simulink model "main"  (R2016a)
settings: Solver=FixedStepAuto  StartTime=0.0  StopTime=inf  FixedStep=0.008  RelTol=1e-3
model workspace: external: MATLAB File initialize_variables_kuramoto.m (data not in the file)
values from neighbouring files (symbols this model uses):
  Angle_offset = [Offset_st, Offset_dev, Offset_rot]    [initialize_variables_kuramoto.m]
  frequency_multiplier = 1    [initialize_variables_kuramoto.m]
  learning_switch = 0    [initialize_variables_matsuoka.m]
  max_dev = 30    [initialize_variables_kuramoto.m]    (also in initialize_variables_matsuoka.m)
  max_rot = 60    [initialize_variables_kuramoto.m]    (also in initialize_variables_matsuoka.m = 90)
  max_stroke = 180    [initialize_variables_kuramoto.m]    (also in initialize_variables_matsuoka.m = 90)
  Offset_st = 0 * gain_st    (= 0)    [initialize_variables_kuramoto.m]
  param_init = [0,0,0,0,0,0 ... (first row only)    [cpg_param_sets.m]    (also in initialize_variables_matsuoka.m)
  param_list = zeros([7,length(Re)*length(A_star)])    [initialize_variables_kuramoto.m]
  step_time = 0.005    [initialize_variables_kuramoto.m]
  w_init = [0 -1.5 0 0 0 0 ... (first row only)    [cpg_param_sets.m]    (also in initialize_variables_matsuoka.m = [0 -2 0 0 -0.1 0)
undefined symbols (not defined in the file or in its folder): frequency, IO3xx, Offset_dev_rot, V
libraries: slrtlib x13, speedgoatlib_fpga x7, simulink x5, powerlib_meascontrol x2
(part 1 of 2)
settings Model: Creator=cedric  LastModifiedBy=kqp5516
settings SolverCC: EnableConcurrentExecution=on
settings DataIOCC: SaveFormat=StructureWithTime  SignalLogging=off  DSMLogging=off  SaveTime=off
settings OptimizationCC: BlockReduction=off  OptimizeBlockIOStorage=off  BufferReuse=off  GlobalBufferReuse=off  ExpressionFolding=off  LocalBlockOutputs=off
settings DebuggingCC: UnderspecifiedInitializationDetection=Classic  MergeDetectMultiDrivingBlocksExec=none  UnconnectedInputMsg=none  UnconnectedOutputMsg=none  UnconnectedLineMsg=none  SFUnexpectedBacktrackingDiag=error  SFNoUnconditionalDefaultTransitionDiag=error
settings HardwareCC: ProdBitPerPointer=32  ProdLargestAtomicFloat=None  ProdWordSize=32  ProdHWDeviceType=Generic->32-bit x86 compatible
settings ModelReferenceCC: PropagateSignalLabelsOutOfModel=off
settings RTWCC: SystemTargetFile=slrt.tlc  TemplateMakefile=slrt_default_tmf  Description=Simulink Real-Time  RTWCompilerOptimization=on
settings SimulinkRealTimeCC: RL32LogTETModifier=off  xPCisModelTimeout=off  xPCModelTimeoutSecs=20
settings ConfigComp: CovMetricSettings=dwe  CovHtmlReporting=off  CovSaveCumulativeToWorkspaceVar=off  CovSaveSingleToWorkspaceVar=off  CovExternalEMLEnable=on

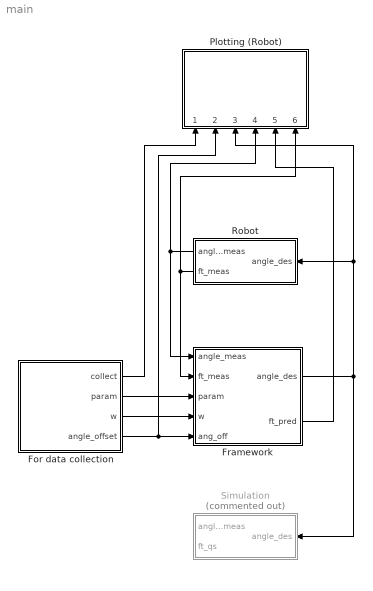
== system main ==
  For data collection : Subsystem
  Framework : Subsystem
  Plotting (Robot) : Subsystem
  Robot : Subsystem
  Simulation : Subsystem  Commented=on
  wires:
  Robot/2(ft_meas) -> Framework/2(ft_meas), Plotting (Robot)/6(ft_meas)
  Robot/1(angle_meas) -> Framework/1(angle_meas), Plotting (Robot)/4(angle_meas)
  Framework/2(ft_pred) -> Plotting (Robot)/5(ft_pred)
  For data collection/4(angle_offset) -> Framework/5(ang_off), Plotting (Robot)/2(angle_offset)
  For data collection/2(param) -> Framework/3(param)
  For data collection/3(w) -> Framework/4(w)
  For data collection/1(collect) -> Plotting (Robot)/1(collect)
  Framework/1(angle_des) -> Plotting (Robot)/3(angle_des), Robot/1(angle_des), Simulation/1(angle_des)

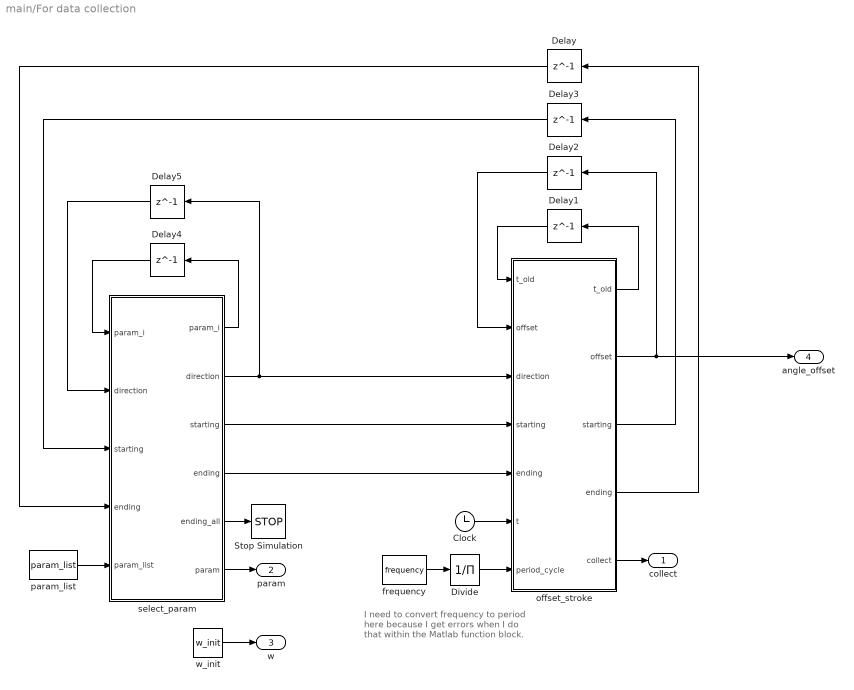
== system main/For data collection ==
  note: I need to convert frequency to period here because I get errors when I do that within the Matlab function block.
  Clock : Clock
  Delay : Delay  DelayLength=1  InitialCondition=0
  Delay1 : Delay  DelayLength=1  InitialCondition=0
  Delay2 : Delay  DelayLength=1  InitialCondition=zeros(3,1)
  Delay3 : Delay  DelayLength=1  InitialCondition=1
  Delay4 : Delay  DelayLength=1  InitialCondition=1
  Delay5 : Delay  DelayLength=1  InitialCondition=1
  Divide : Product  Inputs=/
  Stop Simulation : Stop
  frequency : Constant  Value=frequency
  offset_stroke : MATLAB Function  TreatAsAtomicUnit=on
  param_list : Constant  Value=param_list
  select_param : MATLAB Function  TreatAsAtomicUnit=on
  w_init : Constant  Value=w_init
  collect : Outport
  param : Outport  Port=2
  w : Outport  Port=3
  angle_offset : Outport  Port=4
  wires:
  offset_stroke/2(offset) -> angle_offset/1, Delay2/1
  offset_stroke/4(ending) -> Delay/1
  offset_stroke/1(t_old) -> Delay1/1
  Delay1/1 -> offset_stroke/1("t_old ")
  Delay2/1 -> offset_stroke/2("offset ")
  offset_stroke/3(starting) -> Delay3/1
  Delay3/1 -> select_param/3("starting ")
  Delay/1 -> select_param/4("ending ")
  select_param/3(starting) -> offset_stroke/4("starting ")
  select_param/4(ending) -> offset_stroke/5("ending ")
  select_param/1(param_i) -> Delay4/1
  Delay4/1 -> select_param/1("param_i ")
  select_param/2(direction) -> Delay5/1, offset_stroke/3(direction)
  Delay5/1 -> select_param/2("direction ")
  select_param/5(ending_all) -> Stop Simulation/1
  select_param/6(param) -> param/1
  param_list/1 -> select_param/5(param_list)
  Clock/1 -> offset_stroke/6(t)
  frequency/1 -> Divide/1
  Divide/1 -> offset_stroke/7(period_cycle)
  offset_stroke/5(collect) -> collect/1
  w_init/1 -> w/1

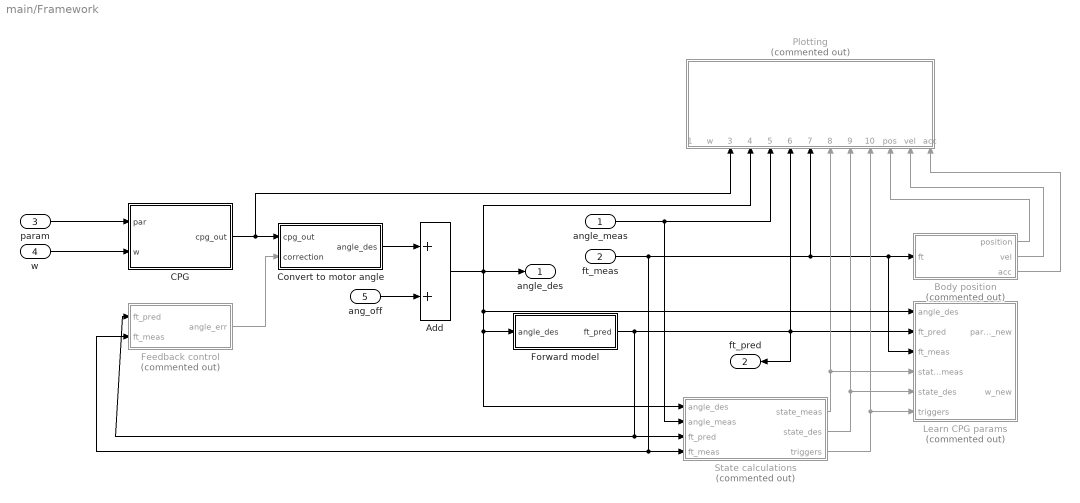
== system main/Framework ==
  angle_meas : Inport
  ft_meas : Inport  Port=2
  param : Inport  Port=3
  w : Inport  Port=4
  ang_off : Inport  Port=5
  Add : Sum
  Body position : Subsystem  Commented=on
  CPG : Subsystem
  Convert to motor angle : Subsystem
  Feedback control : Subsystem  Commented=on
  Forward model : Subsystem
  Learn CPG params : Subsystem  Commented=on
  Plotting : Subsystem  Commented=on
  State calculations : Subsystem  Commented=on
  angle_des : Outport
  ft_pred : Outport  Port=2
  wires:
  CPG/1(cpg_out) -> Plotting/3(cpg_out), Convert to motor angle/1(cpg_out)
  ft_meas/1 -> Plotting/7(ft_meas), Learn CPG params/3(ft_meas), Body position/1(ft), State calculations/4(ft_meas), Feedback control/2(ft_meas)
  State calculations/2(state_des) -> Plotting/9(state_des), Learn CPG params/5(state_des)
  Forward model/1(ft_pred) -> Feedback control/1(ft_pred), State calculations/3(ft_pred), ft_pred/1, Learn CPG params/2(ft_pred), Plotting/6(ft_pred)
  Feedback control/1(angle_err) -> Convert to motor angle/2(correction)
  State calculations/3(triggers) -> Plotting/10(triggers), Learn CPG params/6(triggers)
  Body position/2(vel) -> Plotting/12(vel)
  Body position/1(position) -> Plotting/11(pos)
  Body position/3(acc) -> Plotting/13(acc)
  State calculations/1(state_meas) -> Plotting/8(state_meas), Learn CPG params/4(state_meas)
  angle_meas/1 -> State calculations/2(angle_meas), Plotting/5(angle_meas)
  Convert to motor angle/1(angle_des) -> Add/1
  param/1 -> CPG/1(par)
  w/1 -> CPG/2(w)
  ang_off/1 -> Add/2
  Add/1 -> angle_des/1, Plotting/4(angle_des), State calculations/1(angle_des), Forward model/1(angle_des), Learn CPG params/1(angle_des)

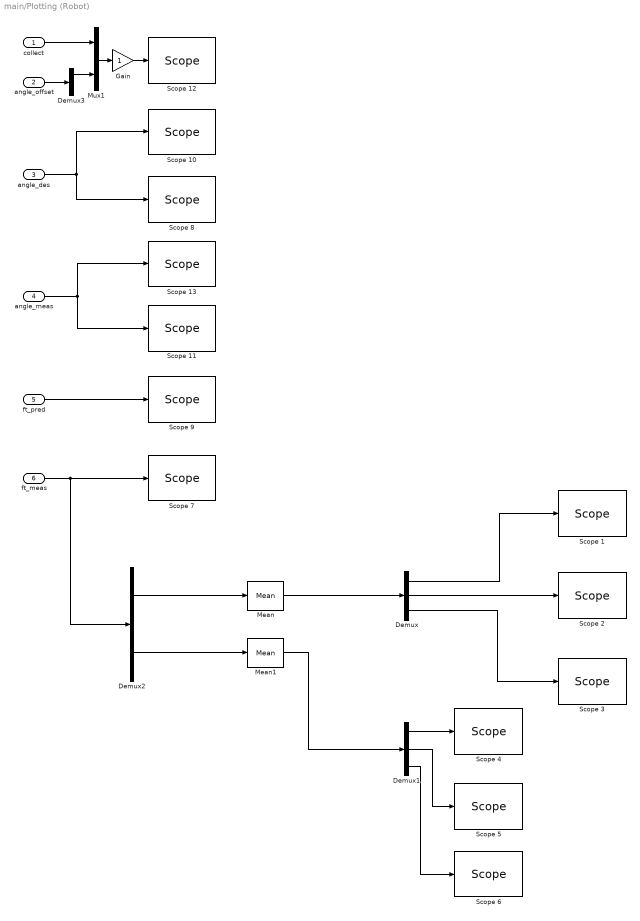
== system main/Plotting (Robot) ==
  collect : Inport
  angle_offset : Inport  Port=2
  angle_des : Inport  Port=3
  angle_meas : Inport  Port=4
  ft_pred : Inport  Port=5
  ft_meas : Inport  Port=6
  Demux : Demux  Outputs=3
  Demux1 : Demux  Outputs=3
  Demux2 : Demux  Outputs=2
  Demux3 : Demux  Outputs=3
  Gain : Gain
  Mean : powerlib_meascontrol/Measurements/Mean  Freq=10  Vinit=0  Ts=0.008
  Mean1 : powerlib_meascontrol/Measurements/Mean  Freq=10  Vinit=0  Ts=0.008
  Mux1 : Mux  Inputs=2
  Scope 1 : slrtlib/Displays and Logging/Scope   scopeno=1  scopetype=Target  autostart=on  viewmode=Graphical rolling  formatstr='%15.6f'  grid=on  ylimits=[0,0]  nosamples=1000  noprepostsamples=0  interleave=5  triggermode=FreeRun  triggersignal=1  trigsignalfromport=off  triggerlevel=0.5  triggerslope=Either  triggerscope=1  triggersample=11000  filename=data.dat  mode=Lazy  writesize=512  autorestart=off  dynamicfilemode=off  maxwritefilesize=512*1024^2
  Scope 10 : slrtlib/Displays and Logging/Scope   scopeno=10  scopetype=File  autostart=on  viewmode=Graphical rolling  formatstr='%15.6f'  grid=on  ylimits=[0,0]  nosamples=10000  noprepostsamples=0  interleave=1  triggermode=FreeRun  triggersignal=1  trigsignalfromport=off  triggerlevel=0.5  triggerslope=Rising  triggerscope=1  triggersample=0  filename=ANGDES_<%>.dat  mode=Lazy  writesize=512  autorestart=on  dynamicfilemode=on  maxwritefilesize=512*1024^2
  Scope 11 : slrtlib/Displays and Logging/Scope   scopeno=11  scopetype=File  autostart=on  viewmode=Graphical rolling  formatstr='%15.6f'  grid=on  ylimits=[0,0]  nosamples=10000  noprepostsamples=0  interleave=1  triggermode=FreeRun  triggersignal=1  trigsignalfromport=off  triggerlevel=0.5  triggerslope=Rising  triggerscope=1  triggersample=0  filename=ANGMEA_<%>.dat  mode=Lazy  writesize=512  autorestart=on  dynamicfilemode=on  maxwritefilesize=512*1024^2
  Scope 12 : slrtlib/Displays and Logging/Scope   scopeno=12  scopetype=File  autostart=on  viewmode=Graphical rolling  formatstr='%15.6f'  grid=on  ylimits=[0,0]  nosamples=10000  noprepostsamples=0  interleave=1  triggermode=FreeRun  triggersignal=1  trigsignalfromport=off  triggerlevel=0.5  triggerslope=Rising  triggerscope=1  triggersample=0  filename=ANGOFF_<%>.dat  mode=Lazy  writesize=512  autorestart=on  dynamicfilemode=on  maxwritefilesize=512*1024^2
  Scope 13 : slrtlib/Displays and Logging/Scope   scopeno=13  scopetype=Target  autostart=on  viewmode=Graphical rolling  formatstr='%15.6f'  grid=on  ylimits=[0,0]  nosamples=1000  noprepostsamples=0  interleave=5  triggermode=FreeRun  triggersignal=1  trigsignalfromport=off  triggerlevel=0.5  triggerslope=Rising  triggerscope=1  triggersample=0  filename=data.dat  mode=Lazy  writesize=512  autorestart=off  dynamicfilemode=off  maxwritefilesize=512*1024^2
  Scope 2 : slrtlib/Displays and Logging/Scope   scopeno=2  scopetype=Target  autostart=on  viewmode=Graphical rolling  formatstr='%15.6f'  grid=on  ylimits=[0,0]  nosamples=1000  noprepostsamples=0  interleave=5  triggermode=FreeRun  triggersignal=1  trigsignalfromport=off  triggerlevel=0.5  triggerslope=Either  triggerscope=1  triggersample=0  filename=data.dat  mode=Lazy  writesize=512  autorestart=off  dynamicfilemode=off  maxwritefilesize=512*1024^2
  Scope 3 : slrtlib/Displays and Logging/Scope   scopeno=3  scopetype=Target  autostart=on  viewmode=Graphical rolling  formatstr='%15.6f'  grid=on  ylimits=[0,0]  nosamples=1000  noprepostsamples=0  interleave=5  triggermode=FreeRun  triggersignal=1  trigsignalfromport=off  triggerlevel=0.5  triggerslope=Rising  triggerscope=1  triggersample=0  filename=data.dat  mode=Lazy  writesize=512  autorestart=off  dynamicfilemode=off  maxwritefilesize=512*1024^2
  Scope 4 : slrtlib/Displays and Logging/Scope   scopeno=4  scopetype=Target  autostart=on  viewmode=Graphical rolling  formatstr='%15.6f'  grid=on  ylimits=[0,0]  nosamples=1000  noprepostsamples=0  interleave=5  triggermode=FreeRun  triggersignal=1  trigsignalfromport=off  triggerlevel=0.5  triggerslope=Rising  triggerscope=1  triggersample=0  filename=data.dat  mode=Lazy  writesize=512  autorestart=off  dynamicfilemode=off  maxwritefilesize=512*1024^2
  Scope 5 : slrtlib/Displays and Logging/Scope   scopeno=5  scopetype=Target  autostart=on  viewmode=Graphical rolling  formatstr='%15.6f'  grid=on  ylimits=[0,0]  nosamples=1000  noprepostsamples=0  interleave=5  triggermode=Software triggering  triggersignal=1  trigsignalfromport=off  triggerlevel=0.5  triggerslope=Rising  triggerscope=1  triggersample=0  filename=data.dat  mode=Lazy  writesize=512  autorestart=off  dynamicfilemode=off  maxwritefilesize=512*1024^2
  Scope 6 : slrtlib/Displays and Logging/Scope   scopeno=6  scopetype=Target  autostart=on  viewmode=Graphical rolling  formatstr='%15.6f'  grid=on  ylimits=[0,0]  nosamples=1000  noprepostsamples=0  interleave=5  triggermode=FreeRun  triggersignal=1  trigsignalfromport=off  triggerlevel=0.5  triggerslope=Rising  triggerscope=1  triggersample=0  filename=data.dat  mode=Lazy  writesize=512  autorestart=off  dynamicfilemode=off  maxwritefilesize=512*1024^2
  Scope 7 : slrtlib/Displays and Logging/Scope   scopeno=7  scopetype=File  autostart=on  viewmode=Graphical rolling  formatstr='%15.6f'  grid=on  ylimits=[0,0]  nosamples=10000  noprepostsamples=0  interleave=1  triggermode=FreeRun  triggersignal=1  trigsignalfromport=off  triggerlevel=0.5  triggerslope=Rising  triggerscope=1  triggersample=0  filename=FTMEA_<%>.dat  mode=Lazy  writesize=512  autorestart=on  dynamicfilemode=on  maxwritefilesize=512*1024^2
  Scope 8 : slrtlib/Displays and Logging/Scope   scopeno=8  scopetype=Target  autostart=on  viewmode=Graphical rolling  formatstr='%15.6f'  grid=on  ylimits=[0,0]  nosamples=1000  noprepostsamples=0  interleave=5  triggermode=FreeRun  triggersignal=1  trigsignalfromport=off  triggerlevel=0.5  triggerslope=Rising  triggerscope=1  triggersample=0  filename=data.dat  mode=Lazy  writesize=512  autorestart=off  dynamicfilemode=off  maxwritefilesize=512*1024^2
  Scope 9 : slrtlib/Displays and Logging/Scope   scopeno=9  scopetype=File  autostart=on  viewmode=Graphical rolling  formatstr='%15.6f'  grid=on  ylimits=[0,0]  nosamples=10000  noprepostsamples=0  interleave=1  triggermode=FreeRun  triggersignal=1  trigsignalfromport=off  triggerlevel=0.5  triggerslope=Rising  triggerscope=1  triggersample=0  filename=FTPRE_<%>.dat  mode=Lazy  writesize=512  autorestart=on  dynamicfilemode=on  maxwritefilesize=512*1024^2
  wires:
  ft_meas/1 -> Demux2/1, Scope 7/1
  Mean/1 -> Demux/1
  Mean1/1 -> Demux1/1
  Demux1/1 -> Scope 4/1
  Demux1/2 -> Scope 5/1
  Demux1/3 -> Scope 6/1
  Demux/1 -> Scope 1/1
  Demux/2 -> Scope 2/1
  Demux/3 -> Scope 3/1
  Demux2/1 -> Mean/1
  Demux2/2 -> Mean1/1
  angle_des/1 -> Scope 10/1, Scope 8/1
  angle_meas/1 -> Scope 13/1, Scope 11/1
  ft_pred/1 -> Scope 9/1
  collect/1 -> Mux1/1
  angle_offset/1 -> Demux3/1
  Demux3/1 -> Mux1/2
  Mux1/1 -> Gain/1
  Gain/1 -> Scope 12/1

== system main/Robot ==
  angle_des : Inport
  Analog Force Signal : Subsystem
  Control : Subsystem
  Serial Setup : speedgoatlib_fpga/Serial/Serial Setup  id=1  channel=[1 6]  bitrate_configuration=Simple  bitrate=[1000000]  bitrate_effective=[1e6, 1e6]  bitrate_error=[0, 0]  base_clock=[75000000, 75000000]  divider=[5, 5]  cpr=[1, 1]  tcr=[15, 15]  parity=No parity  nb_data_bits=[8]  nb_stop_bits=[1]  rs485_half_duplex=on  board=IO323  pciSlot=-1
  Setup : speedgoatlib_fpga/Setup/Setup  board=IO323  id=1  frontIO=None  rearIO=IO3xx-22  bitstreamFile=speedgoat_IO323_22_CI_01532  ProgSpiFlash=off  ProgBPIFlash=off  pciSlot=-1  PullRPort0=pull-up 3.3V  VioPort0=3.3V  PullRPort1=pull-up 3.3V  VioPort1=3.3V  PullRPort2=pull-up 3.3V  VioPort2=3.3V  PullRPort3=pull-up 3.3V  VioPort3=3.3V  PullRPort4=pull-up 3.3V  VioPort4=3.3V  PullRPort5=pull-up 3.3V  VioPort5=3.3V  PullRPort6=pull-up 3.3V  VioPort6=3.3V  PullRPort15=pull-up 3.3V  PullRPort31=pull-up 3.3V  PullRPort47=pull-up 3.3V  PullRPort63=pull-up 3.3V
  angle_meas : Outport
  ft_meas : Outport  Port=2
  wires:
  angle_des/1 -> Control/1(reference)
  Control/1(ang_meas) -> angle_meas/1
  Analog Force Signal/1(ft) -> ft_meas/1

== system main/Simulation ==
  angle_des : Inport  PortDimensions=3
  Add : Sum
  Band-Limited White Noise : simulink/Sources/Band-Limited White Noise  Commented=on  Cov=[0.0001,0.0001,0.0001]  Ts=0.008  seed=[23341,438,1376]
  Demux : Demux  Commented=on  Outputs=3
  QS Model : Subsystem
  Scope : Scope  Commented=on  NumInputPorts=3
  angle_meas : Outport
  ft_qs : Outport  Port=2
  wires:
  angle_des/1 -> Add/1, angle_meas/1
  QS Model/1(ft_qs) -> ft_qs/1
  Add/1 -> QS Model/1(angle_des)
  Band-Limited White Noise/1 -> Add/2, Demux/1
  Demux/1 -> Scope/1
  Demux/2 -> Scope/2
  Demux/3 -> Scope/3

== system main/Framework/Body position ==
  ft : Inport  PortDimensions=6
  Equations of motion : MATLAB Function  TreatAsAtomicUnit=on
  Integrator : Integrator  InitialCondition=zeros(3,1)
  Integrator1 : Integrator  InitialCondition=zeros(3,1)
  position : Outport
  vel : Outport  Port=2
  acc : Outport  Port=3
  wires:
  ft/1 -> Equations of motion/1(ft)
  Equations of motion/1(acc) -> acc/1, Integrator/1
  Integrator/1 -> Integrator1/1, vel/1
  Integrator1/1 -> position/1

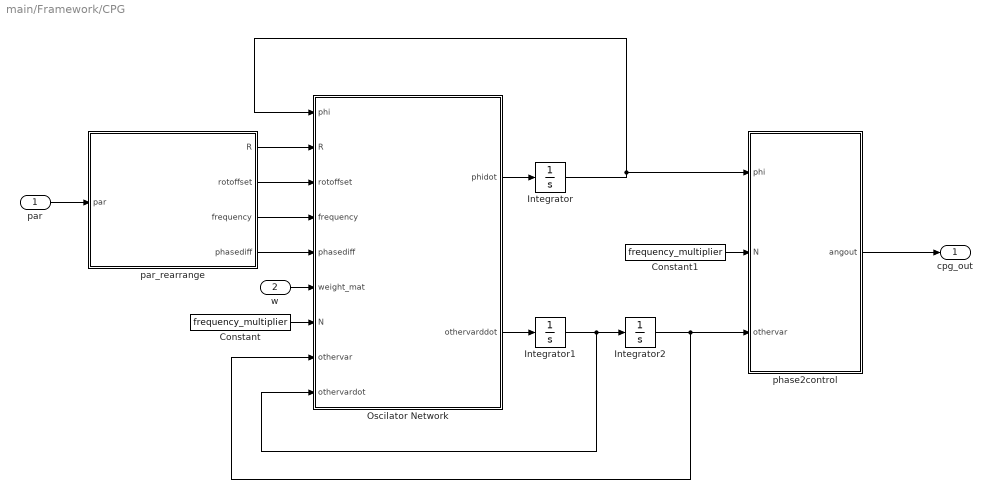
== system main/Framework/CPG ==
  par : Inport
  w : Inport  Port=2
  Constant : Constant  Value=frequency_multiplier
  Constant1 : Constant  Value=frequency_multiplier
  Integrator : Integrator
  Integrator1 : Integrator
  Integrator2 : Integrator
  Oscilator Network : MATLAB Function  TreatAsAtomicUnit=on
  par_rearrange : MATLAB Function  TreatAsAtomicUnit=on
  phase2control : MATLAB Function  TreatAsAtomicUnit=on
  cpg_out : Outport
  wires:
  par/1 -> par_rearrange/1(par)
  Oscilator Network/1(phidot) -> Integrator/1
  par_rearrange/1(R) -> Oscilator Network/2(R)
  Oscilator Network/2(othervarddot) -> Integrator1/1
  Integrator1/1 -> Integrator2/1, Oscilator Network/9(othervardot)
  Integrator2/1 -> Oscilator Network/8(othervar), phase2control/3(othervar)
  par_rearrange/3(frequency) -> Oscilator Network/4(frequency)
  par_rearrange/4(phasediff) -> Oscilator Network/5(phasediff)
  phase2control/1(angout) -> cpg_out/1
  par_rearrange/2(rotoffset) -> Oscilator Network/3(rotoffset)
  Integrator/1 -> Oscilator Network/1(phi), phase2control/1(phi)
  Constant/1 -> Oscilator Network/7(N)
  Constant1/1 -> phase2control/2(N)
  w/1 -> Oscilator Network/6(weight_mat)

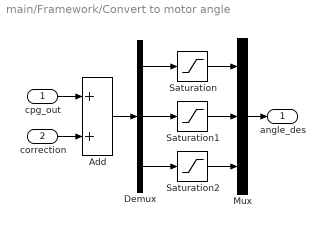
== system main/Framework/Convert to motor angle ==
  cpg_out : Inport  Interpolate=off
  correction : Inport  Port=2
  Add : Sum
  Demux : Demux  Outputs=3
  Mux : Mux  Inputs=3
  Saturation : Saturate  UpperLimit=max_stroke  LowerLimit=-max_stroke
  Saturation1 : Saturate  UpperLimit=max_dev  LowerLimit=-max_dev
  Saturation2 : Saturate  UpperLimit=max_rot  LowerLimit=-max_rot
  angle_des : Outport
  wires:
  Mux/1 -> angle_des/1
  Demux/2 -> Saturation1/1
  Demux/3 -> Saturation2/1
  Demux/1 -> Saturation/1
  Saturation/1 -> Mux/1
  Saturation2/1 -> Mux/3
  Saturation1/1 -> Mux/2
  correction/1 -> Add/2
  cpg_out/1 -> Add/1
  Add/1 -> Demux/1

== system main/Framework/Feedback control ==
  ft_pred : Inport
  ft_meas : Inport  Port=2
  Delay2 : Delay  DelayLength=1
  Delay3 : Delay  DelayLength=1
  MATLAB Function : MATLAB Function  TreatAsAtomicUnit=on
  angle_err : Outport
  wires:
  ft_meas/1 -> Delay2/1
  ft_pred/1 -> Delay3/1
  MATLAB Function/1(angle_correction) -> angle_err/1
  Delay2/1 -> MATLAB Function/2(ft_meas)
  Delay3/1 -> MATLAB Function/1(ft_pred)

== system main/Framework/Forward model ==
  angle_des : Inport
  QS Model : Subsystem
  ft_pred : Outport
  wires:
  angle_des/1 -> QS Model/1(angle_des)
  QS Model/1(ft_qs) -> ft_pred/1

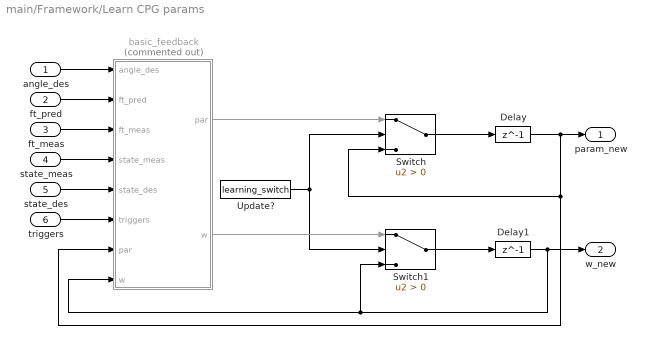
== system main/Framework/Learn CPG params ==
  angle_des : Inport  PortDimensions=3
  ft_pred : Inport  Port=2  PortDimensions=6
  ft_meas : Inport  Port=3  PortDimensions=6
  state_meas : Inport  Port=4
  state_des : Inport  Port=5
  triggers : Inport  Port=6
  Delay : Delay  DelayLength=1  InitialCondition=param_init
  Delay1 : Delay  DelayLength=1  InitialCondition=w_init
  Switch : Switch  Criteria=u2 > Threshold
  Switch1 : Switch  Criteria=u2 > Threshold
  Update? : Constant  Value=learning_switch
  basic_feedback : MATLAB Function  Commented=on  TreatAsAtomicUnit=on
  param_new : Outport
  w_new : Outport  Port=2
  wires:
  ft_meas/1 -> basic_feedback/3(ft_meas)
  ft_pred/1 -> basic_feedback/2(ft_pred)
  angle_des/1 -> basic_feedback/1(angle_des)
  Update?/1 -> Switch/2, Switch1/2
  Switch/1 -> Delay/1
  basic_feedback/1(par) -> Switch/1
  basic_feedback/2(w) -> Switch1/1
  Switch1/1 -> Delay1/1
  triggers/1 -> basic_feedback/6(triggers)
  state_meas/1 -> basic_feedback/4(state_meas)
  state_des/1 -> basic_feedback/5(state_des)
  Delay/1 -> Switch/3, basic_feedback/7("par "), param_new/1
  Delay1/1 -> Switch1/3, basic_feedback/8("w "), w_new/1

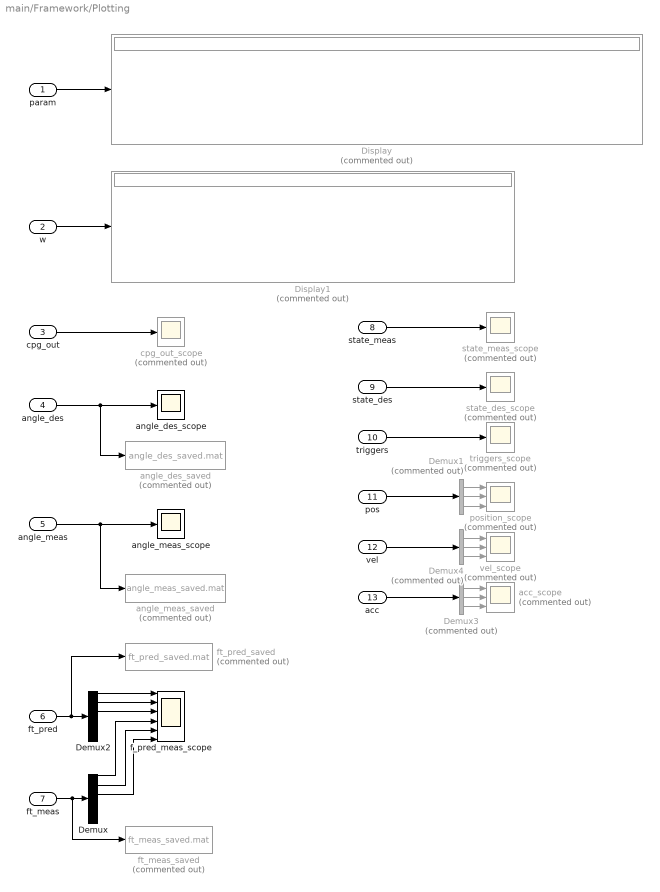
== system main/Framework/Plotting ==
  param : Inport
  w : Inport  Port=2
  cpg_out : Inport  Port=3
  angle_des : Inport  Port=4
  angle_meas : Inport  Port=5
  ft_pred : Inport  Port=6
  ft_meas : Inport  Port=7
  state_meas : Inport  Port=8
  state_des : Inport  Port=9
  triggers : Inport  Port=10
  pos : Inport  Port=11
  vel : Inport  Port=12
  acc : Inport  Port=13
  Demux : Demux  Outputs=6
  Demux1 : Demux  Commented=on  Outputs=3
  Demux2 : Demux  Outputs=6
  Demux3 : Demux  Commented=on  Outputs=3
  Demux4 : Demux  Commented=on  Outputs=3
  Display : Display  Commented=on
  Display1 : Display  Commented=on
  acc_scope : Scope  Commented=on  NumInputPorts=3
  angle_des_saved : ToFile  Commented=on  Filename=angle_des_saved.mat  MatrixName=angle_des_saved
  angle_des_scope : Scope
  angle_meas_saved : ToFile  Commented=on  Filename=angle_meas_saved.mat  MatrixName=angle_meas_saved
  angle_meas_scope : Scope
  cpg_out_scope : Scope  Commented=on
  f_pred_meas_scope : Scope  NumInputPorts=6
  ft_meas_saved : ToFile  Commented=on  Filename=ft_meas_saved.mat  MatrixName=ft_meas_saved
  ft_pred_saved : ToFile  Commented=on  Filename=ft_pred_saved.mat  MatrixName=ft_pred_saved  SaveFormat=Timeseries
  position_scope : Scope  Commented=on  NumInputPorts=3
  state_des_scope : Scope  Commented=on
  state_meas_scope : Scope  Commented=on
  triggers_scope : Scope  Commented=on
  vel_scope : Scope  Commented=on  NumInputPorts=3
  wires:
  Demux1/1 -> position_scope/1
  Demux1/2 -> position_scope/2
  Demux1/3 -> position_scope/3
  Demux3/1 -> acc_scope/1
  Demux3/2 -> acc_scope/2
  Demux3/3 -> acc_scope/3
  Demux4/1 -> vel_scope/1
  Demux4/2 -> vel_scope/2
  Demux4/3 -> vel_scope/3
  pos/1 -> Demux1/1
  vel/1 -> Demux4/1
  acc/1 -> Demux3/1
  ft_meas/1 -> ft_meas_saved/1, Demux/1
  ft_pred/1 -> ft_pred_saved/1, Demux2/1
  cpg_out/1 -> cpg_out_scope/1
  angle_meas/1 -> angle_meas_saved/1, angle_meas_scope/1
  angle_des/1 -> angle_des_saved/1, angle_des_scope/1
  triggers/1 -> triggers_scope/1
  state_meas/1 -> state_meas_scope/1
  param/1 -> Display/1
  w/1 -> Display1/1
  state_des/1 -> state_des_scope/1
  Demux2/1 -> f_pred_meas_scope/1
  Demux2/2 -> f_pred_meas_scope/2
  Demux2/3 -> f_pred_meas_scope/3
  Demux/1 -> f_pred_meas_scope/4
  Demux/2 -> f_pred_meas_scope/5
  Demux/3 -> f_pred_meas_scope/6

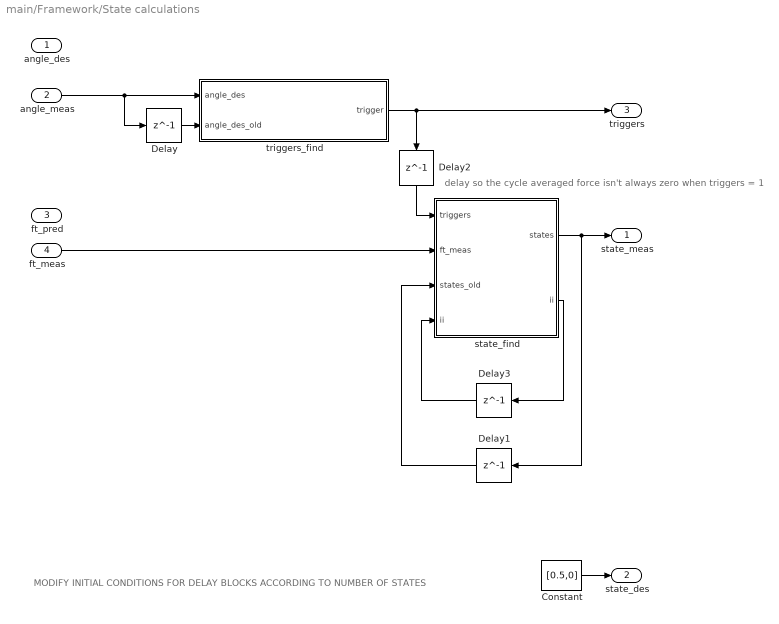
== system main/Framework/State calculations ==
  note: MODIFY INITIAL CONDITIONS FOR DELAY BLOCKS ACCORDING TO NUMBER OF STATES
  note: delay so the cycle averaged force isn't always zero when triggers = 1
  angle_des : Inport
  angle_meas : Inport  Port=2
  ft_pred : Inport  Port=3
  ft_meas : Inport  Port=4
  Constant : Constant  Value=[0.5,0]
  Delay : Delay  DelayLength=1
  Delay1 : Delay  DelayLength=1  InitialCondition=zeros(2,1)
  Delay2 : Delay  DelayLength=1  InitialCondition=zeros(2,1)
  Delay3 : Delay  DelayLength=1  InitialCondition=zeros(2,1)
  state_find : MATLAB Function  TreatAsAtomicUnit=on
  triggers_find : MATLAB Function  TreatAsAtomicUnit=on
  state_meas : Outport
  state_des : Outport  Port=2
  triggers : Outport  Port=3
  wires:
  angle_meas/1 -> Delay/1, triggers_find/1(angle_des)
  Delay/1 -> triggers_find/2(angle_des_old)
  triggers_find/1(trigger) -> triggers/1, Delay2/1
  state_find/1(states) -> Delay1/1, state_meas/1
  Delay1/1 -> state_find/3(states_old)
  ft_meas/1 -> state_find/2(ft_meas)
  Constant/1 -> state_des/1
  Delay2/1 -> state_find/1(triggers)
  state_find/2(ii) -> Delay3/1
  Delay3/1 -> state_find/4("ii ")

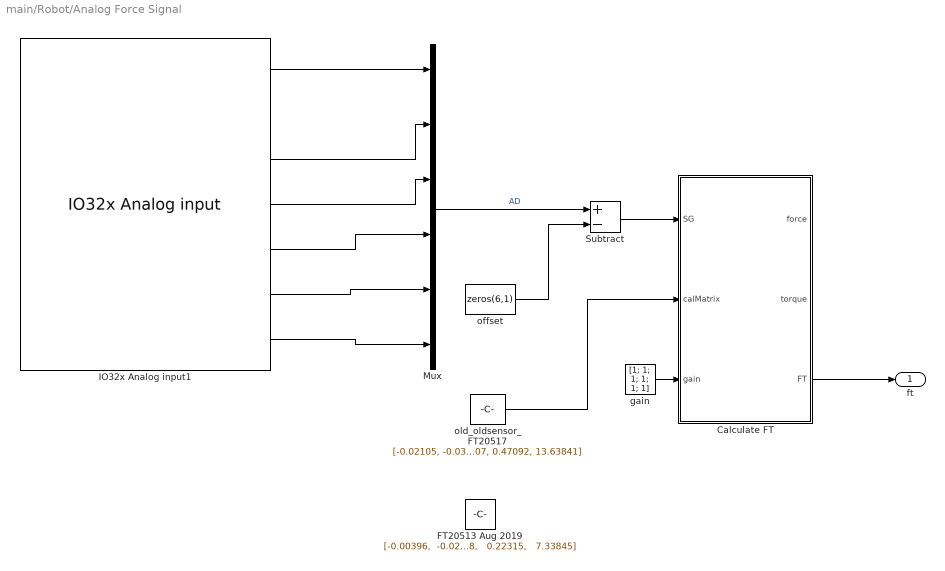
== system main/Robot/Analog Force Signal ==
  Calculate FT : MATLAB Function  TreatAsAtomicUnit=on
  FT20513 Aug 2019 : Constant  Value="[-0.00396,  -0.02626,  -0.00148,  -1.65041,   0.05372,   1.61165;-0.00147,   2.05926,  -0.01141,  -0.98505,  -0.01508,  -0.91035; 1.88736,  -0.01982,   1.94791,  -0.03636,   1.85673,  -0.02132;-0.06688,  12.60494,  10.47872,  -6.15582, -10.64754,  -5.52308; -11.71646,   0.24827,   6.66712,   9.99714,   6.01967,  -9.86076;0.06228,   7.36314,  -0.02169,   7.00298,   0.22315,   7.33845]"  VectorParams1D=off
  IO32x Analog input1 : speedgoatlib_fpga/Analog IO/IO32x Analog input  id=1  pciSlot=-1  board=IO323  ts=step_time  ADC1_chan=[]  ADC1_range=± 5.12 [V]  ADC1_diff=Differential  ADC1_Trigger=Initiator  ADC1_Seq=on  ADC2_chan=[]  ADC2_range=± 5.12 [V]  ADC2_diff=Differential  ADC2_Trigger=Initiator  ADC2_Seq=on  ADC3_chan=[1,2,3,4]  ADC3_range=± 5.12 [V]  ADC3_diff=Differential  ADC3_Trigger=Initiator  ADC3_Seq=on  ADC4_chan=[1,2,3]  ADC4_range=± 5.12 [V]  ADC4_diff=Differential  ADC4_Trigger=Initiator  ADC4_Seq=on
  Mux : Mux  Inputs=6
  Subtract : Sum  Inputs=+-
  gain : Constant  Value=[1; 1; 1; 1; 1; 1]
  offset : Constant  Value=zeros(6,1)
  old_oldsensor_FT20517 : Constant  Value=|
      | [-0.02105, -0.03378, 0.01181, -3.41616, 0.10427, 3.24450;
      | 0.07611, 3.90936, -0.05439, -1.96630, -0.05318, -1.85101;
      | 3.69041, -0.12722, 4.15582, -0.02600, 3.89697, 0.01945;
      | 0.45716, 23.52815, 22.84137, -12.03285, -22.23834, -11.17787;
      | -23.42535, 1.16989, 13.35133, 20.38198, 11.64139 -19.51054;
      | 0.19958, 14.59346, 0.13476, 14.65607, 0.47092, 13.63841]
  ft : Outport
  wires:
  IO32x Analog input1/1 -> Mux/1
  IO32x Analog input1/5 -> Mux/4
  IO32x Analog input1/6 -> Mux/5
  gain/1 -> Calculate FT/3(gain)
  IO32x Analog input1/4 -> Mux/3
  IO32x Analog input1/3 -> Mux/2
  IO32x Analog input1/7 -> Mux/6
  offset/1 -> Subtract/2
  Calculate FT/3(FT) -> ft/1
  Subtract/1 -> Calculate FT/1(SG)
  Mux/1 -> Subtract/1  "AD"
  old_oldsensor_FT20517/1 -> Calculate FT/2(calMatrix)

== system main/Robot/Control ==
  note: The Serial block performs both reading and writing operations on the motors.
  reference : Inport  PortDimensions=[1,3]
  Chart : Stateflow chart  TreatAsAtomicUnit=on
  Delay2 : Delay  DelayLength=1
  Serial : Subsystem
  ang_meas : Outport
  wires:
  reference/1 -> Chart/2(reference)
  Chart/1(control) -> Serial/1(control)
  Chart/2(write_type) -> Serial/2(write_type)
  Serial/1(angle) -> ang_meas/1, Delay2/1
  Delay2/1 -> Chart/1(position)

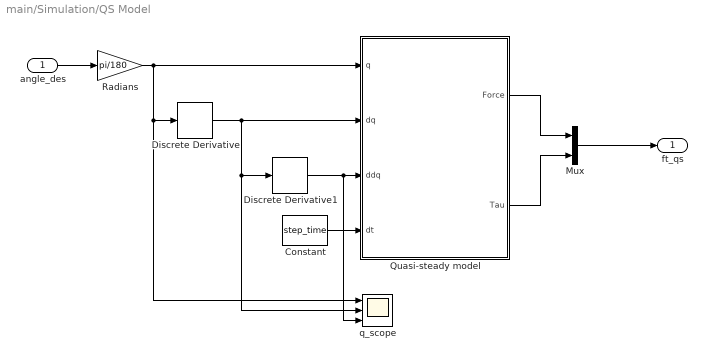
== system main/Simulation/QS Model ==
  angle_des : Inport  PortDimensions=3
  Constant : Constant  Value=step_time
  Discrete Derivative : simulink/Discrete/Discrete Derivative  gainval=1.0  ICPrevScaledInput=0.0  OutMin=[]  OutMax=[]  OutDataType=fixdt(1, 16)  OutScaling=2^-10  DoSatur=off
  Discrete Derivative1 : simulink/Discrete/Discrete Derivative  gainval=1.0  ICPrevScaledInput=0.0  OutMin=[]  OutMax=[]  OutDataType=fixdt(1, 16)  OutScaling=2^-10  DoSatur=off
  Mux : Mux  Inputs=2
  Quasi-steady model : MATLAB Function  TreatAsAtomicUnit=on
  Radians : Gain  Gain=pi/180
  q_scope : Scope  NumInputPorts=3
  ft_qs : Outport
  wires:
  angle_des/1 -> Radians/1
  Discrete Derivative/1 -> Quasi-steady model/2(dq), Discrete Derivative1/1, q_scope/2
  Mux/1 -> ft_qs/1
  Quasi-steady model/1(Force) -> Mux/1
  Discrete Derivative1/1 -> q_scope/3, Quasi-steady model/3(ddq)
  Constant/1 -> Quasi-steady model/4(dt)
  Radians/1 -> Discrete Derivative/1, q_scope/1, Quasi-steady model/1(q)
  Quasi-steady model/2(Tau) -> Mux/2

== system main/Framework/Forward model/QS Model ==
  angle_des : Inport  PortDimensions=3
  Constant : Constant  Value=step_time
  Discrete Derivative : simulink/Discrete/Discrete Derivative  gainval=1.0  ICPrevScaledInput=0.0  OutMin=[]  OutMax=[]  OutDataType=fixdt(1, 16)  OutScaling=2^-10  DoSatur=off
  Discrete Derivative1 : simulink/Discrete/Discrete Derivative  gainval=1.0  ICPrevScaledInput=0.0  OutMin=[]  OutMax=[]  OutDataType=fixdt(1, 16)  OutScaling=2^-10  DoSatur=off
  Mux : Mux  Inputs=2
  Quasi-steady model : MATLAB Function  TreatAsAtomicUnit=on
  Radians : Gain  Gain=pi/180
  q_scope : Scope  NumInputPorts=3
  ft_qs : Outport
  wires:
  angle_des/1 -> Radians/1
  Discrete Derivative/1 -> Quasi-steady model/2(dq), Discrete Derivative1/1, q_scope/2
  Mux/1 -> ft_qs/1
  Quasi-steady model/1(Force) -> Mux/1
  Discrete Derivative1/1 -> q_scope/3, Quasi-steady model/3(ddq)
  Constant/1 -> Quasi-steady model/4(dt)
  Radians/1 -> Discrete Derivative/1, q_scope/1, Quasi-steady model/1(q)
  Quasi-steady model/2(Tau) -> Mux/2

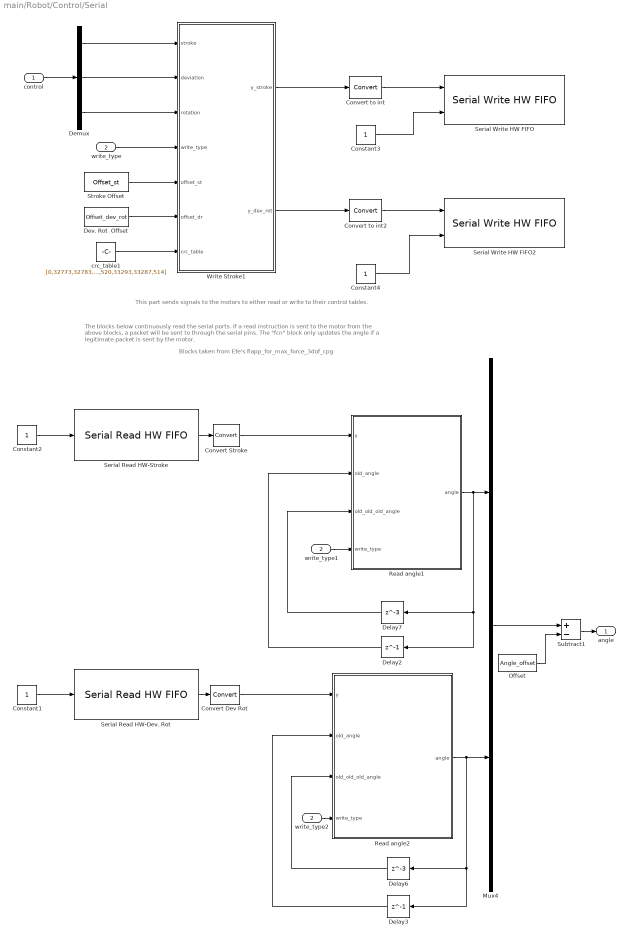
== system main/Robot/Control/Serial ==
  note: Blocks taken from Efe's flapp_for_max_force_3dof_cpg
  note: The blocks below continuously read the serial ports. If a read instruction is sent to the motor from the above blocks, a packet will be sent to through the serial pins. The "fcn" block only updates the angle if a legitimate packet is sent by the motor.
  note: This part sends signals to the motors to either read or write to their control tables.
  control : Inport
  write_type : Inport  Port=2
  " Offset" : Constant  Value=Angle_offset  VectorParams1D=off
  Constant{1..4} (4 alike) : Constant  OutDataTypeStr=Inherit: Inherit via back propagation
  Convert Dev Rot : DataTypeConversion
  Convert Stroke : DataTypeConversion
  Convert to int : DataTypeConversion
  Convert to int2 : DataTypeConversion
  Delay2 : Delay  DelayLength=1  SampleTime=step_time
  Delay3 : Delay  DelayLength=1  SampleTime=step_time
  Delay6 : Delay  DelayLength=3  SampleTime=step_time
  Delay7 : Delay  DelayLength=3  SampleTime=step_time
  Demux : Demux  Outputs=3
  Dev. Rot  Offset : Constant  Value=Offset_dev_rot  VectorParams1D=off
  Mux4 : Mux  Inputs=2
  Read angle1 : MATLAB Function  TreatAsAtomicUnit=on
  Read angle2 : MATLAB Function  TreatAsAtomicUnit=on
  Serial Read HW-Dev. Rot : speedgoatlib_fpga/Serial/Serial Read HW FIFO  id=1  channel=6  board=IO323  nb_data_bits=8  pciSlot=-1  ts=step_time
  Serial Read HW-Stroke : speedgoatlib_fpga/Serial/Serial Read HW FIFO  id=1  channel=1  board=IO323  nb_data_bits=8  pciSlot=-1  ts=step_time
  Serial Write HW FIFO : speedgoatlib_fpga/Serial/Serial Write HW FIFO  id=1  channel=1  board=IO323  tx_fifo_mode=Halt model on buffer overflow  nb_data_bits=8  pciSlot=-1  ts=step_time
  Serial Write HW FIFO2 : speedgoatlib_fpga/Serial/Serial Write HW FIFO  id=1  channel=6  board=IO323  tx_fifo_mode=Halt model on buffer overflow  nb_data_bits=8  pciSlot=-1  ts=step_time
  Stroke Offset : Constant  Value=Offset_st
  Subtract1 : Sum  Inputs=+-
  Write Stroke1 : MATLAB Function  TreatAsAtomicUnit=on
  crc_table1 : Constant  Value=[0,32773,32783,10,32795,30,20,32785,32819,54,60,32825,40,32813,32807,34,32867,102,108,32873,120,32893,32887,114,80,32853,32863,90,32843,78,68,32833,32963,198,204,32969,216,32989,32983,210,240,33013,33023,250,33003,238,228,32993,160,32933,32943,170,32955,190,180,32945,32915,150,156,32921,136,32909,32903,130,33155,390,396,33161,408,33181,33175,402,432,33205,33215,442,33195,430,420,33185,480,33253,33263,490,33275,510,500,33265,33235,470,476,33241,456,33229,33223,450,320,33093,33103,330,33115,350,340,33105,33139,374,380,33145,360,33133,33127,354,33059,294,300,33065,312,33085,33079,306,272,33045,33055,282,33035,270,260,33025,33539,774,780,33545,792,33565,33559,786,816,33589,33599,826,33579,814,804,33569,864,33637,33647,874,33659,894,884,33649,33619,854,860,33625,840,33613,33607,834,960,33733,33743,970,33755,990,980,33745,33779,1014,1020,33785,1000,33773,33767,994,33699,934,940,33705,952,33725,33719,946,912,33685,33695,922,33675,910,900,33665,640,33413,33423,650,33435,670,660,33425,33459,694,700,33465,680,33453,33447,674,33507,742,748,33513,760,33533,33527,754,720,33493,33503,730,33483,718,708,33473,33347,582,588,33353,600,33373,33367,594,624,33397,33407,634,33387,622,612,33377,544,33317,33327,554,33339,574,564,33329,33299,534,540,33305,520,33293,33287,514]  OutDataTypeStr=Inherit: Inherit via back propagation
  write_type1 : InportShadow  Port=2
  write_type2 : InportShadow  Port=2
  angle : Outport
  wires:
  Constant3/1 -> Serial Write HW FIFO/2
  Convert to int2/1 -> Serial Write HW FIFO2/1
  Constant4/1 -> Serial Write HW FIFO2/2
  control/1 -> Demux/1
  Convert to int/1 -> Serial Write HW FIFO/1
  Demux/1 -> Write Stroke1/1(stroke)
  Demux/2 -> Write Stroke1/2(deviation)
  Demux/3 -> Write Stroke1/3(rotation)
  write_type/1 -> Write Stroke1/4(write_type)
  crc_table1/1 -> Write Stroke1/7(crc_table)
  Write Stroke1/1(y_stroke) -> Convert to int/1
  Write Stroke1/2(y_dev_rot) -> Convert to int2/1
  Stroke Offset/1 -> Write Stroke1/5(offset_st)
  Dev. Rot  Offset/1 -> Write Stroke1/6(offset_dr)
  Convert Stroke/1 -> Read angle1/1(y)
  Constant1/1 -> Serial Read HW-Dev. Rot/1
  Convert Dev Rot/1 -> Read angle2/1(y)
  Read angle1/1(angle) -> Delay2/1, Delay7/1, Mux4/1
  Constant2/1 -> Serial Read HW-Stroke/1
  Delay2/1 -> Read angle1/2(old_angle)
  Delay3/1 -> Read angle2/2(old_angle)
  Delay6/1 -> Read angle2/3(old_old_old_angle)
  Delay7/1 -> Read angle1/3(old_old_old_angle)
  Read angle2/1(angle) -> Delay3/1, Delay6/1, Mux4/2
  Mux4/1 -> Subtract1/1
  " Offset"/1 -> Subtract1/2
  write_type1/1 -> Read angle1/4(write_type)
  write_type2/1 -> Read angle2/4(write_type)
  Subtract1/1 -> angle/1
  Serial Read HW-Stroke/1 -> Convert Stroke/1
  Serial Read HW-Dev. Rot/1 -> Convert Dev Rot/1

== matlab function main/Framework/CPG/par_rearrange ==
  data: par input; R output; rotoffset output; frequency output; phasediff output
function [R, rotoffset, frequency, phasediff] = par_rearrange(par)

R          = par(1:3);
rotoffset  = par(4);
phasediff  = ([0; par(5:6)])*pi/180;
frequency  = par(7);

== matlab function main/Framework/CPG/phase2control ==
  data: phi input; angout output; N input; othervar input
function angout  = phase2control(phi, N, othervar)

% angout = theta in paper = oscillating set-point in radians

r      = othervar(1:3,1);
x      = othervar(4:6,1);

angout = nan(3,1);
angout(1) = r(1)*sin(phi(1));
angout(2) = r(2)*sin(N*phi(2));
angout(3) = r(3)*sin(phi(3));

angout = angout + x;

== stateflow chart main/Robot/Control/Chart ==
  state INIT
    entry:
    write_type = 0;
    during:
    write_type = 1;
    control = position;
  state Move
    state RW_SCHEDULING [parallel]
      settings: executionOrder=1
      state READ
        entry:
        write_type = 1;
      state WRITE
        entry:
        write_type = 2;
      (default) -> READ
      WRITE -> READ
      READ -> WRITE
    state Controller [parallel]
      settings: executionOrder=2
      state Move
        entry:
        control = position;
        during:
        error    = reference-position;
        control = control + (abs(error) > 0.2).* [1,1,0.5].*min(max(-0.08,error*0.015),0.08);
        stage = 1;
        exit:
        control = reference;
      state Stay
        during:
        stage = 2;
        exit:
        control=position;
      (default) -> Move.Controller.Move
      Move.Controller.Move -> Stay : [norm(reference-position)<2]
      Stay -> Move.Controller.Move : [norm(reference-position)>3]
  note: Does it keep switching between read and write cycles?
  note: What is the control variable? It seems like it's the goal angle value.
  note: The controller makes the motors "stay" at a control signal as long as error is <=2?
  (default) -> INIT
  INIT -> Move : after(1,sec)
  data: control output; write_type output; position input; reference input; error local; stage output

== matlab function main/Robot/Analog Force Signal/Calculate FT ==
  data: SG input; force output; calMatrix input; gain input; torque output; FT output
function [force, torque, FT]  = calFT(SG,calMatrix,gain)
%#codegen

for i=1:6
    calMatrix(:,i) = calMatrix(:,i)/gain(i);
end
% SG1=SG;
FT = calMatrix * (SG);

force = FT(1:3);% Unit: N
torque = FT(4:6);% Unit: N*mm

end

== matlab function main/Framework/CPG/Oscilator Network ==
  data: phi input; R input; rotoffset input; frequency input; phasediff input; weight_mat input; phidot output; N input; othervar input; othervarddot output; othervardot input
function [phidot, othervarddot] = oscillators(phi, R, rotoffset, frequency, phasediff, weight_mat, N, othervar, othervardot)
% Translation to "Controlling swimming and crawling in a fish robot using a
%   central pattern generator" CPG

% phi = phase of oscillations
% r and R = current and desired amplitude of oscillations (m and M in Efe's
%           paper)
% x and X = current and desired offset of oscillations
% f = frequency = desired frequency of oscillations (same for all motors)
% ax and ar = decay rates for the critically damped amplitude dynamics
% w = weight_mat = coupling weight between oscillators i and j
% psi = phase bias between oscillators i and j
%       matrix contains desired phase difference between stroke and other
%       two motors

% othervar is r and x as 1 variable - each have dimension 3, for 3 motors
% ref is similarly R and X as 1 var
% same for a

ar = 5*ones(3,1);
ax = 5*ones(3,1);                  % amplitude convergence rate
a  = [ar;ax];

X      = [0;0;rotoffset];
ref    = [R;X];
Nvec           = [1; N; 1];
% weight_map     = [0, 1 , 1;        % connection weight           
%                   1, 0 , 0;         % see Efe paper p. 3 for non-zero
%                   1, 0 , 0];
%               
% weight_adjust  = 2;
% 
% weight_mat  = weight_map*weight_adjust*2*pi*frequency/length(R); 

phasebias   = phasediff./Nvec;      % ???


phasebias_mat  = [phasebias(1),  phasebias(2), phasebias(3);    % why is element 11 not 0? turns out phasebias(1) = 0 always
                 -phasebias(2), 0            , 0;               % aren't we supposed to use phi to get this?
                 -phasebias(3), 0            , 0;];
             
             
% phidot eqn missing r inside the sum?
phidot        = 2*pi*frequency + sum((weight_mat) .* sin(ones(length(phi),1)*phi'-phi*ones(1,length(phi))-phasebias_mat),2);
othervarddot  = a.*((a/4).*(ref-othervar)-othervardot);

== matlab function main/Framework/Feedback control/MATLAB Function ==
  data: ft_pred input; ft_meas input; angle_correction output
function angle_correction = feedback(ft_pred,ft_meas)
%#codegen

ft_err = ft_meas - ft_pred;
gain_rot = 1.1;

angle_correction = zeros(3,1);

% change angle of attack depending on movement direction
if motor_angle(3) > 0 % flexor
    angle_correction(3) = -gain_rot*ft_err(1);
    
elseif motor_angle(3) < 0 % extensor
    angle_correction(3) = +gain_rot*ft_err(1);
end

== matlab function main/Framework/Learn CPG params/basic_feedback ==
  data: angle_des input; ft_pred input; ft_meas input; state_meas input; state_des input; triggers input; par input; w input; par output; w output
function [par,w] = feedback(angle_des,ft_pred,ft_meas,state_meas,state_des,triggers,par,w)

% Inputs:
%   state_des = desired values for states like velocity, acc, etc.
%   triggers = array of 0 and 1 corresponding to each desired goal
%               if 1, then check if the corresponding goal is being met and
%               change params accordingly

% N = length(w);
R          = par(1:3);
rotoffset  = par(4);
phasediff  = ([0; par(5:6)]);
frequency  = par(7);

%% desired cycle averaged values - feedforward
% only adjust cpg params if triggers are activated

% lift
if triggers(1) == 1
    gain_lift = 1.5;
    cycle_averaged_lift = state_meas(1) - state_des(1);
    
    if cycle_averaged_lift > 0
        frequency = frequency / gain_lift;% * cycle_averaged_lift;
    elseif cycle_averaged_lift < 0
        frequency = frequency * gain_lift;% * cycle_averaged_lift);
    end
end

% x - fore/aft
if triggers(2) == 1
    % reduce stroke in opposite direction of where its high
    % flexor goes back, extensor goes forward
    step_x = 5;
    cycle_averaged_x = state_meas(2) - state_des(2);
    
    if cycle_averaged_x > 0
        rotoffset = rotoffset + step_x;
    elseif cycle_averaged_x < 0
        rotoffset = rotoffset - step_x;
    end
end

% possible problems with this approach:
%   if different goals interfere with each other, then feedback could be
%       detrimental

%% internal model predictions vs measured - feedback
% ACTUALLY SCRATCH THIS IDEA - CORRECT MOTOR SIGNAL DIRECTLY USING FEEDBACK

% % map ft_err_pred to cpg params
% ft_err_pred = ft_meas - ft_pred;
% 
% % max Feed
% % max_Feed_stroke = 30;
% % max_Feed_dev = 20;
% max_Feed_rot = 30;
% gain_Feed_rot = 10;
% 
% % adjust angle of attack if measured force in x is different than predicted
% % change extensor or flexor feed depending on phase
% if motor_angle(3)>0 % flexor
%     Feed(6) = 0;
%     % change angle of attack depending on part of the stroke cycle
% %     if motor_angle(1)<0
% %         Feed(5) = -gain_Feed_rot*ft_err_pred(1);
% %     elseif motor_angle(1)>0
% %         Feed(5) = +gain_Feed_rot*ft_err_pred(1);
% %     end
%     Feed(5) = -gain_Feed_rot*ft_err_pred(1);
%     
% elseif motor_angle(3)<0 % extensor
%     Feed(5) = 0;
%     Feed(6) = +gain_Feed_rot*ft_err_pred(1);
% 
% else
%     Feed(5) = 0;
%     Feed(6) = 0;
% end
% 
%  % limit Feed
% if abs(Feed(5)) > max_Feed_rot
%     Feed(5) = Feed(5)/abs(Feed(5)) * max_Feed_rot;
% end
% if abs(Feed(6)) > max_Feed_rot
%     Feed(6) = Feed(6)/abs(Feed(6)) * max_Feed_rot;
% end

%% update param
par(1:3) = R;
par(4) = rotoffset;
par(5:6) = phasediff(2:3);
par(7) = frequency;

== matlab function main/Framework/Body position/Equations of motion ==
  data: ft input; acc output
function acc  = newtons(ft)
% only takes position in account
% may need to convert ft to body frame if ft is in wing frame

m = 1; % point mass
forces = ft(1:3);

acc = forces/m;

== matlab function main/Framework/Forward model/QS Model/Quasi-steady model ==
  data: q input; Force output; dq input; ddq input; dt input; Tau output
%#codegen

%%%%%%%%%%%%%%%%%%%%%%%%%%%%%%%%%%%%%%%%%%%%%%%%%%%%%%%%%%%%%%%%%%%%%%%%%%%
%%%%%%%%%%%%%%   Aerodynamic forces and moments calculator   %%%%%%%%%%%%%%
%%%%%%%%%%%%%%%%%%%%%%%%%%%%%%%%%%%%%%%%%%%%%%%%%%%%%%%%%%%%%%%%%%%%%%%%%%%

% This program calcuates the aerodynamic forces and moments generated by a
% flapping wing

% The aerodynamic forces and torques at each wing blade element is
% evaluated by aerodynamics

function [Force,Tau] =Aerodynamic_Force_Torque(q,dq,ddq,dt)
    
% q=[stroke angle;deviation angle; rotation angle]
% dq= dq/dt;
% ddq= dq/dt;

%% Define variables 
    
%     omega_l            % Anular velocity of wing in global frame
%     omega_l_d          % Anular Acc of Right wing in body frame
%     Rcl                %(Rcl* vector_follower=vector_base //    follwer is Wing and Global is base)

    [Rcl,omega_l,omega_l_d] = AngKinZXY(q,dq,ddq);
    %% Hinge parameters

%     lhz  --> Stroke Hinge offset in stroke frame
%     lhx  --> Deviation Hinge offset in deviation frame
%     lhy  --> Rotation Hinge offset in Rotation frame

% Change these parameter according to your setup 
    lhz = [0;0;-0.15];
    lhx = [0;0;0];
    lhy = [0;0.05;0];
    

    vel_h_l = rotz(q(1))*( cross([0;0;dq(1)],lhz) + rotx(q(2))*( cross([dq(2);0;0],lhx) + roty(q(3))*cross([0;dq(3);0],lhy) ));       % Velocity of Hinge in global frame
    
    %% Transform to wing frame
 
    omega_l=Rcl\omega_l;
    omega_l_d=Rcl\omega_l_d;
    vel_h_l  =  Rcl\vel_h_l;
    % transform from global to wing frame



    %%
    rho = 826;      % air density  1.2041(20C) 1.1839(25C)  1.1644(30C)  1.455(35C)
    NumBlade = 10;         % spatial resolution: number of blade elements


% Change these parameter according to your setup 
    Rw = 0.18;          % wing length
    AR = 3;             % Aspect Ratio
    chord = Rw/AR;        % chord length
        

    %% step through a wing span: spanwise location: 0<i<=1
    
    % Initialise variables
    F_t = zeros(3,1);
    Tau_t = zeros(3,1);

    
    for j = 1:NumBlade
        i = j/NumBlade;
        
        % obtain local aerodynamic force/torques in Hinge frame
        % omega_l and omega_r; omega_l_d and omega_r_d in body frame
        % omega_b and vel_h are in global frame
        % omega_b and vel_h have to be expressed differently for left and right wings
        
        % Force and Torque at each blade elements
        [Fi_t, Taui_t] = aerodynamics_left(omega_l,vel_h_l,omega_l_d,i,dt,Rw,chord, NumBlade,rho);

       %% Summation along wing span
       % integrate along wing span and transform to stroke plane frame
       F_t = F_t +  Fi_t;    
       Tau_t =  Tau_t +  Taui_t;


    end

    % All the forces and torque obtain are in Left and Right Wing frame
    % Tranform them to Hinge frame 
 
    Force=Rcl*F_t;

    Tau=Rcl*Tau_t ;
    
end





%% %%%%%%%%%%%%%%%%%%%%%%%%%%%%%%%%%%%%%%%%%%%%%%%%%%%%%%%%%%%%%%%%%%%%%%%%
%  %%%%%%%%%%%%%%%%%%%%%%%%%%%%%%%%%%%%%%%%%%%%%%%%%%%%%%%%%%%%%%%%%%%%%%%%
%  %%%%%%%%%%%%%%%%%%%%%%%%%%%%%%%%%%%%%%%%%%%%%%%%%%%%%%%%%%%%%%%%%%%%%%%%

%-------------------------------------------------------------------
%----------   Aerodynamics Module For Wing  -------------------
%-------------------------------------------------------------------

% This function takes in wing kinematics (angle/velocity/accleration) and body velocity
% and calcuates the aerodynamic force/torque created by each wing blade (w.r.t local blade coordinate frame)
% then convert it to Hinge frame

% torques are with respect to the wing hinges.

% all the values are w.r.t to local blade coordinate frame (different from stroke
% plane frame), except original input of vel_h, omega_w, omege_w_d and omega_b are in stroke plane frame

% wing coordinate frame: (left wing) x points to ventral side (normal to the wing surface), y from wing base to tip, z from trailing to leading edge

% export tip velocity and span-averaged angle of attack

function [Fi, Taui] = aerodynamics_left(omega_w,vel_h, omega_w_d,i,dt,Rw,chord, NumBlade,rho)
 

%% blade-element analysis 
    % i=location of the blade element
    rle = -i*Rw;  % spanwise location of the blade element
    
    % local wing blade velocity 
    vle = cross(omega_w,[0 rle 0]') + vel_h;            % local leading edge velocity in wing frame
    vle(2)=0;                                                   % igonre radial velocity component                                    

    % angular velocity of the last time instant, here omega_b is assumed to be constant
    omega_wLI = omega_w-omega_w_d*dt;
    
    % velocity of the last time instant
    
    vleLI = cross(omega_wLI,[0 rle 0]') + vel_h;                        
    vleLI(2)=0;                                                 % igonre radial velocity component   
    
    % linear accleration along xw direction
    acc_xw = (vle(1)-vleLI(1))/dt;
    % angualr acceleration about yw direction
    omega_yw_dot = omega_w_d(2);

    
    %% Direction of blade velocity
    % get the direction of the local blade velocity
    if norm(vle) ~= 0
        dir_vle = vle/norm(vle)  ;                 % local leading edge velocity direction vector in left wing frame
        alpha = abs(atan(dir_vle(1)/dir_vle(3)));  
    else
        dir_vle = [0;0;0];
        alpha = 0;  
    end
    
    % local drag direction
    dir_drag = -dir_vle;  
    dir_drag(2)=0; 
    % local lift direction
    dir_lift = roty( -sign( vle(1)) *pi/2 ) * dir_vle;         
    % local angle of attack (consider X as imaginary axis and Z as real axis, only 1st and 2nd quadrants are considered)

    %%  wing sectional lift and drag due to translational force components
    % (2*CD(alpha_l)*rle/R) is sectional drag coefficient
    q   = 0.5*rho*(norm(vle))^2;
    FDi = q*(CD_hu(alpha)) * chord * (Rw/NumBlade)*dir_drag;  
    FLi = q*(CL_hu(alpha)) * chord * (Rw/NumBlade)*dir_lift;

    % center of pressure (translational component)
    r_cof_trans = chord*(0.82*abs(alpha)/pi+0.05);

    %%  wing sectional lift and drag due to rotational force components
    
    % Change these parameter according to your setup 
    x_rot = 0.453;  % rotational axis, 0 corresponds to leading edge
    
    Circulation_rot = pi*(0.75-x_rot) * chord^2 * omega_w(2);  % cirulcation over a wing chord
    F_rot_i = (Rw/NumBlade)*[ rho * Circulation_rot * norm(vle), 0, 0]';
    % center of pressure (rotational component)

    r_cof_rot = x_rot*chord;  % old
    
    %%  wing sectional lift and drag due to added-mass force components
    cr = (-x_rot+0.5)*chord; % distance between center of wing rotation and mid-point of wing chord
    % coefficient of virtual mass
    lamda_x = pi*rho*(0.5*chord)^2;
    lamda_xo = -pi*rho*(0.5*chord)^2*cr;

    % added mass force components
    F_addx_i = lamda_x*acc_xw - lamda_xo*omega_yw_dot;

    % force vector due to added mass
    F_add_i = (Rw/NumBlade)*[F_addx_i, 0,0]'; 

    % center of pressure (added mass component)
    r_cof_add = x_rot*chord;   

    %% summation of all force components and convert them to Hinge frame
    % sum  wing local force vectors
    Fi =  (FDi - FLi -F_add_i - F_rot_i);

    % sum wing local torque vectors
    Taui =(cross([0 rle r_cof_trans]',FDi-FLi) + cross([0 rle r_cof_add]',-F_add_i)+cross([0 rle r_cof_rot]',-F_rot_i));  

 

end


function [R,Omega,alpha] = AngKinZXY(q,dq,ddq)

R=rotz(q(1))*rotx(q(2))*roty(q(3));

w2=[0;0;dq(1)] + rotz(q(1)) * ([dq(2);0;0] );
w1=[0;0;dq(1)] ;

Omega=[0;0;dq(1)]...
    + rotz(q(1)) * [dq(2);0;0] ...
    + rotz(q(1)) * rotx(q(2))*[0;dq(3);0];

alpha=[0;0;ddq(1)]...
    + S(w1)*rotz(q(1)) * [dq(2);0;0] +  rotz(q(1)) * [ddq(2);0;0] ...
    + S(w2)*(rotz(q(1)) * rotx(q(2)))*[0;dq(3);0] +(rotz(q(1)) * rotx(q(2)))*[0;ddq(3);0];
end

function Sw = S(w)
%%%%%%%%%%%%%%%%%%%%%%%%%%%%%%%%%%%%%%%%%%%%%%%%%%%%%%%%%%%%%%%%%%%%%%%%%%%
% % Calculate Cross Product matrix
% % cross(w,R)--> Sw  *  R
%%%%%%%%%%%%%%%%%%%%%%%%%%%%%%%%%%%%%%%%%%%%%%%%%%%%%%%%%%%%%%%%%%%%%%%%%%%
Sw = [0 -w(3) w(2);
    w(3) 0 -w(1);
    -w(2) w(1) 0];
end

function CL = CL_hu(alpha)
alphadeg = alpha *180/pi;       % to degrees
CL = 0.245 + 1.63*sin((2.34*alphadeg - 6.3)*pi/180);
end

% rotation matrices
% b/c code generation doesn't seem to support built-in ones
function CD = CD_hu(alpha)
alphadeg = alpha *180/pi;       % to degrees
CD = 1.88-1.70*cos((2.27*alphadeg - 10.66)*pi/180);
end

function R = rotx(angle)
R = [1 0 0;
    0 cos(angle) -sin(angle);
    0 sin(angle) cos(angle)];
end

function R = roty(angle)
R = [cos(angle) 0 sin(angle);
    0 1 0;
    -sin(angle) 0 cos(angle)];
end

function R = rotz(angle)
R = [cos(angle) -sin(angle) 0;
    sin(angle) cos(angle) 0;
    0 0 1];
end
